simulink model "Task_35"  (R2022b)
settings: Solver=VariableStepAuto  StartTime=0.0  StopTime=10.0  RelTol=1e-3
settings Model: Creator=Abanob_Sameh  LastModifiedBy=Abanob_Sameh

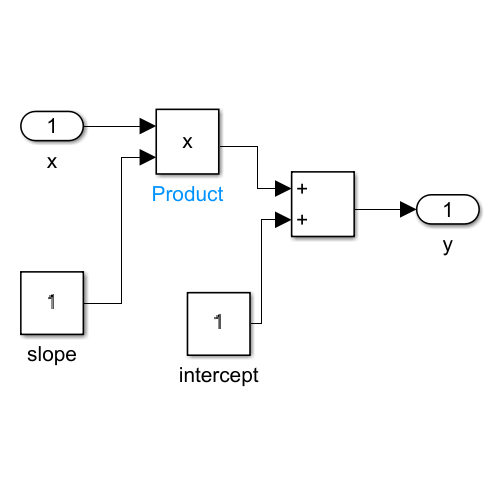
[thumbnail: Simulink's stored preview of the top-level diagram]
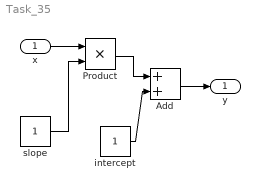
== system Task_35 ==
  x : Inport
  Add : Sum
  Product : Product
  intercept : Constant
  slope : Constant
  y : Outport
  wires:
  x/1 -> Product/1
  intercept/1 -> Add/2
  slope/1 -> Product/2
  Product/1 -> Add/1
  Add/1 -> y/1
